simulink model "transformerparamether"  (R2020b)
settings: Solver=VariableStepAuto  StartTime=0.0  StopTime=10.0  RelTol=1e-3
libraries: powerlib x13, powerlib_meascontrol x7
settings Model: Creator=admin  LastModifiedBy=admin

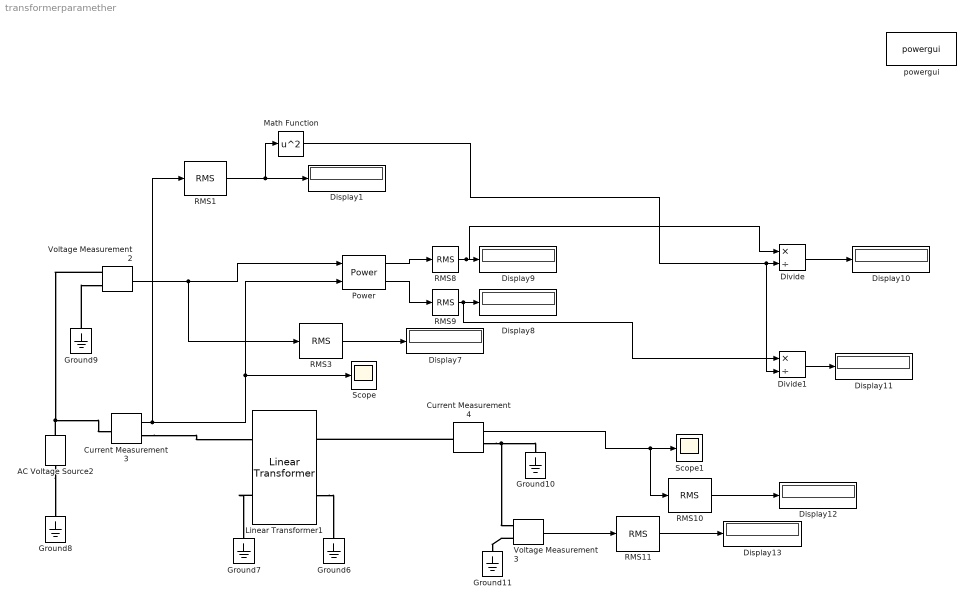
== system transformerparamether ==
  AC Voltage Source2 : powerlib/Electrical Sources/AC Voltage Source  Amplitude=150*sqrt(2)  Phase=0  Frequency=50  SampleTime=0  Measurements=Voltage  BusType=swing  Pref=10e3  Qref=0  Qmin=-inf  Qmax=+inf
  Current Measurement3 : powerlib/Measurements/Current Measurement  PhasorSimulation=off  OutputType=Complex  PSBequivalent=0
  Current Measurement4 : powerlib/Measurements/Current Measurement  PhasorSimulation=off  OutputType=Complex  PSBequivalent=0
  Display{1,7..13} (8 alike) : Display
  Divide : Product  Inputs=*/
  Divide1 : Product  Inputs=*/
  Ground{6..11} (6 alike) : powerlib/Elements/Ground  LConnTagsString=a
  Linear Transformer1 : powerlib/Elements/Linear Transformer  UNITS=SI  NominalPower=[250e6 50 ]  winding1=[2400 4.3218 0.45856]  winding2=[240 0.7938 0.084225]  ThreeWindings=off  winding3=[3.15e+05 0.7938 0.084225]  RmLm=[1.0805e+06 2866]  Measurements=None  DataType=on
  Math Function : Math  Operator=square  SaturateOnIntegerOverflow=on
  Power : powerlib_meascontrol/Measurements/Power  Freq=60  Vinit=[1, 0]  Iinit=[1, 0]  Ts=0
  RMS{1,3,8..11} (6 alike) : powerlib_meascontrol/Measurements/RMS  TrueRMS=on  Freq=50  RMSInit=0  Ts=0
  Scope : Scope
  Scope1 : Scope
  Voltage Measurement2 : powerlib/Measurements/Voltage Measurement  PhasorSimulation=off  OutputType=Complex  PSBequivalent=0
  Voltage Measurement3 : powerlib/Measurements/Voltage Measurement  PhasorSimulation=off  OutputType=Complex  PSBequivalent=0
  powergui : powerlib/powergui  Priority=1  SimulationMode=Continuous  SampleTime=50e-6  frequency=60  Iterations=50  frequencyindice=50  Pbase=100e6  ErrMax=1e-4  UnitsV=kV  UnitsW=MW  buscounter=0  FunctionMessages=off  echomessages=off  EnableUseOfTLC=off  CurrentSourceSwitches=off  DisableSnubberDevices=off  DisableRonSwitches=off  DisableVfSwitches=off  DisplayEquations=off  AutomaticDiscreteSolvers=off  SolverType=Tustin/Backward Euler (TBE)  Interpol=off  ExternalGateDelay=off  methode=off  Ts=100  x0status=blocks  SPID=on  SwTol=0  HookPort=off  NonlinearTolerance=1e-4  nMaxIteration=100  ContinueOnMaxIteration=off  RestoreLinks=warning  ResistiveCurrentMeasurement=off  Frange=[0:2:500]  Ylog=off  Xlog=on  ShowGrid=off  save=off  variable=ZData  structure=0  ZoomFFT=off  StartTime=0.0  cycles=1  DisplayStyle=1  fundamental=60  FreqAxis=off  MaxFrequency=1000  frequencyindicesteady=1  RmsSteady=1  display=off
  wires:
  Voltage Measurement2/1 -> RMS3/1, Power/1
  Current Measurement3/1 -> RMS1/1, Scope/1, Power/2
  RMS1/1 -> Display1/1, Math Function/1
  RMS3/1 -> Display7/1
  Power/1 -> RMS8/1
  Power/2 -> RMS9/1
  Math Function/1 -> Divide1/2, Divide/2
  RMS8/1 -> Divide/1, Display9/1
  RMS9/1 -> Divide1/1, Display8/1
  Divide/1 -> Display10/1
  Divide1/1 -> Display11/1
  Current Measurement4/1 -> RMS10/1, Scope1/1
  RMS10/1 -> Display12/1
  Voltage Measurement3/1 -> RMS11/1
  RMS11/1 -> Display13/1
  connections:
  AC Voltage Source2/LConn1 -- Ground8/LConn1
  Voltage Measurement2/LConn1 -- AC Voltage Source2/RConn1 -- Current Measurement3/LConn1
  Current Measurement3/RConn1 -- Linear Transformer1/LConn1
  Linear Transformer1/LConn2 -- Ground7/LConn1
  Linear Transformer1/RConn2 -- Ground6/LConn1
  Ground9/LConn1 -- Voltage Measurement2/LConn2
  Current Measurement4/LConn1 -- Linear Transformer1/RConn1
  Current Measurement4/RConn1 -- Voltage Measurement3/LConn1 -- Ground10/LConn1
  Voltage Measurement3/LConn2 -- Ground11/LConn1
